simulink model "Simulink_PowerFactor_Calculations_Example"  (R2021a)
settings: Solver=ode23tb  StartTime=0.0  StopTime=0.1  MaxStep=50e-6  RelTol=1e-4  EnableMultiTasking=on
PreLoadFcn:
  | Ts=50e-6;
libraries: spsPowerLib x1
settings Model: Creator=The MathWorks, Inc.  LastModifiedBy=EREN-PC
settings SolverCC: AlgebraicLoopSolver=TrustRegion
settings DataIOCC: LimitDataPoints=on  SaveFormat=Array  ReturnWorkspaceOutputs=off
settings OptimizationCC: ExpressionDepthLimit=2147483647  LifeSpan=inf
settings DebuggingCC: UnderspecifiedInitializationDetection=Classic  MergeDetectMultiDrivingBlocksExec=none  FcnCallInpInsideContextMsg=warning  SignalLabelMismatchMsg=warning  StateNameClashWarn=warning  SFUnexpectedBacktrackingDiag=warning  SFNoUnconditionalDefaultTransitionDiag=warning  SFExecutionAtInitializationDiag=none  SFMachineParentedDataDiag=warning  ArithmeticOperatorsInVariantConditions=warning
settings HardwareCC: ProdBitPerPointer=32  ProdBitPerSizeT=32  ProdBitPerPtrDiffT=32  ProdLargestAtomicFloat=None  ProdIntDivRoundTo=Undefined  ProdEndianess=Unspecified  ProdWordSize=32  ProdHWDeviceType=32-bit Generic
settings ModelReferenceCC: PropagateSignalLabelsOutOfModel=off
settings SFSimCC: SimUseLocalCustomCode=off  CustomCodeUndefinedFunction=UseInterfaceOnly
settings RTWCC: RTWUseLocalCustomCode=off
settings CodeAppCC: StateflowObjectComments=on
settings GRTTargetCC: TargetLangStandard=C89/C90 (ANSI)  CombineOutputUpdateFcns=off  GRTInterface=on
settings ConfigComp: CovMetricSettings=dw  CovSaveCumulativeToWorkspaceVar=on  CovSaveSingleToWorkspaceVar=on  CovExternalEMLEnable=off  CovSFcnEnable=off

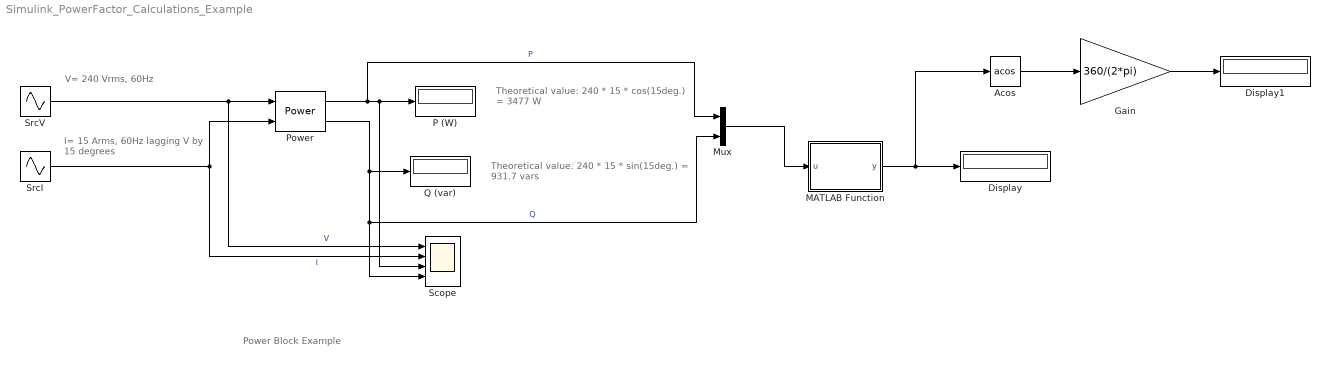
== system Simulink_PowerFactor_Calculations_Example ==
  note: Power Block Example
  note: V= 240 Vrms, 60Hz
  note: I= 15 Arms, 60Hz
      | lagging V by 15 degrees
  note: Theoretical value:
      | 240 * 15 * cos(15deg.) = 3477 W
  note: Theoretical value:
      | 240 * 15 * sin(15deg.) = 931.7 vars
  Acos : Trigonometry  Operator=acos
  Display : Display
  Display1 : Display
  Gain : Gain  Gain=360/(2*pi)
  MATLAB Function : MATLAB Function  TreatAsAtomicUnit=on
  Mux : Mux  Inputs=2
  P (W) : Display
  Power : spsPowerLib/Power  Freq=60  Vinit=[240*sqrt(2) 0]  Iinit=[15*sqrt(2) -15]  Ts=Ts
      settings: SourceProductBaseCode=PS
  Q (var) : Display
  Scope : Scope  NumInputPorts=4
  SrcI : Sin  Amplitude=15*sqrt(2)  Frequency=2*pi*60  Phase=-15 * (pi/180)  SampleTime=Ts
  SrcV : Sin  Amplitude=240*sqrt(2)  Frequency=2*pi*60  SampleTime=Ts
  wires:
  SrcV/1 -> Power/1, Scope/1  "V"
  SrcI/1 -> Scope/2, Power/2  "I"
  Power/1 -> Mux/1, P (W)/1, Scope/3  "P"
  Power/2 -> Q (var)/1, Mux/2, Scope/4  "Q"
  Mux/1 -> MATLAB Function/1(u)
  MATLAB Function/1(y) -> Acos/1, Display/1
  Acos/1 -> Gain/1
  Gain/1 -> Display1/1

== matlab function Simulink_PowerFactor_Calculations_Example/MATLAB Function ==
  data: u input; y output
function y = fcn(u)

y = u(1)/(sqrt((u(1)*u(1))+u(2)*u(2)));
